simulink model "Diferensial"  (R2023b)
settings: Solver=VariableStepAuto  StartTime=0.0  StopTime=10.0  RelTol=1e-3
settings Model: Creator=Eye Patch  LastModifiedBy=Eye Patch

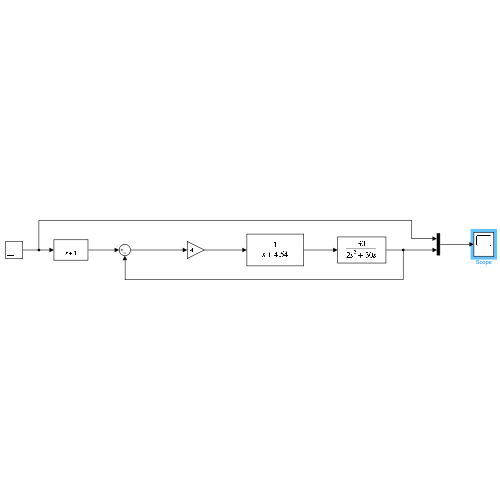
[thumbnail: Simulink's stored preview of the top-level diagram]
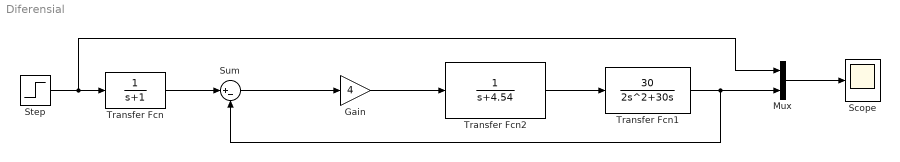
== system Diferensial ==
  Gain : Gain  Gain=4
  Mux : Mux  Inputs=2
  Scope : Scope
  Step : Step  SampleTime=0
  Sum : Sum  Inputs=|+-
  Transfer Fcn : TransferFcn  Denominator=[1 1]
  Transfer Fcn1 : TransferFcn  Numerator=[30]  Denominator=[2 30 0]
  Transfer Fcn2 : TransferFcn  Denominator=[1 4.54]
  wires:
  Transfer Fcn1/1 -> Mux/2, Sum/2
  Gain/1 -> Transfer Fcn2/1
  Transfer Fcn2/1 -> Transfer Fcn1/1
  Step/1 -> Mux/1, Transfer Fcn/1
  Transfer Fcn/1 -> Sum/1
  Sum/1 -> Gain/1
  Mux/1 -> Scope/1
